simulink model "buckConverter"  (R2021a)
settings: Solver=VariableStepAuto  StartTime=0.0  StopTime=1  RelTol=1e-3
model workspace (MAT data in the model file):
  C = Simulink.Parameter
  C.Value = 0.01
  C.DataType = 'double'
  C.Dimensions = [1 1]
  L = Simulink.Parameter
  L.Value = 0.01
  L.DataType = 'double'
  L.Dimensions = [1 1]
  R = Simulink.Parameter
  R.Value = 10
  R.DataType = 'double'
  R.Dimensions = [1 1]
  Vin = Simulink.Parameter
  Vin.Value = 100
  Vin.DataType = 'double'
  Vin.Dimensions = [1 1]
libraries: spsSeriesRLCBranchLib x3, spsCurrentMeasurementLib x2, spsDCVoltageSourceLib x1, spsDiodeLib x1, spsIGBTLib x1, spsVoltageMeasurementLib x1, spspowerguiLib x1
settings Model: Creator=User  LastModifiedBy=User

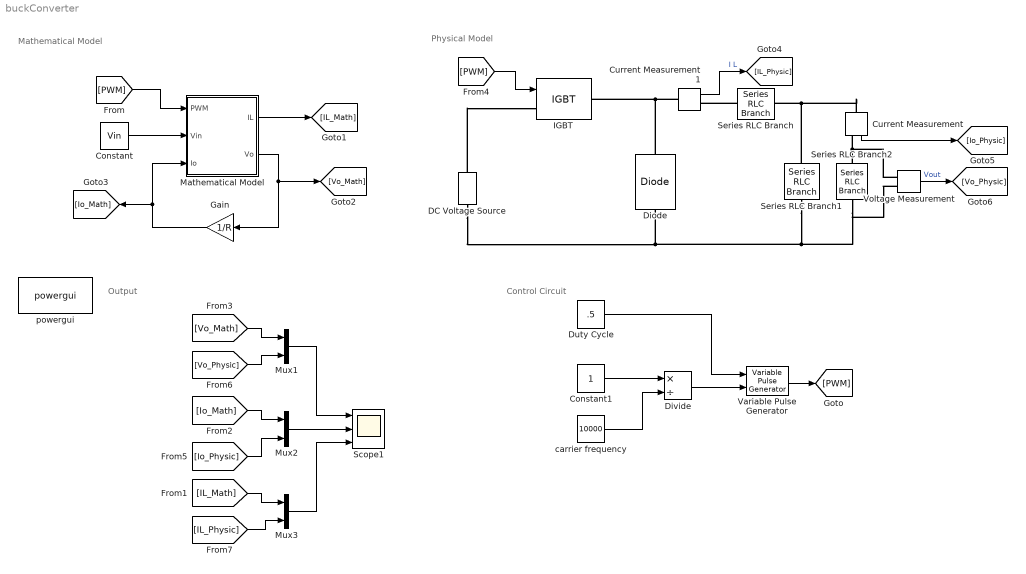
== system buckConverter ==
  note: Output
  note: Mathematical Model
  note: Physical Model
  note: Control Circuit
  Constant : Constant  Value=Vin
  Constant1 : Constant
  Current Measurement : spsCurrentMeasurementLib/Current Measurement  PhasorSimulation=off  OutputType=Complex  PSBequivalent=0
  Current Measurement1 : spsCurrentMeasurementLib/Current Measurement  PhasorSimulation=off  OutputType=Complex  PSBequivalent=0
  DC Voltage Source : spsDCVoltageSourceLib/DC Voltage Source  Amplitude=Vin  Measurements=None
  Diode : spsDiodeLib/Diode  Ron=0.001  Lon=0  Vf=0.8  IC=0  UseSnubber=0  Rs=500  Cs=250e-9  Measurements=off
  Divide : Product  Inputs=*/
  Duty Cycle : Constant  Value=.5
  Gain : Gain  Gain=1/R
  IGBT : spsIGBTLib/IGBT  Ron=0.001  Lon=0  Vf=1  Tf=1e-6  Tt=2e-6  IC=0  Rs=1e5  Cs=inf  Measurements=off
  Mathematical Model : Subsystem
  Mux1 : Mux  Inputs=2
  Mux2 : Mux  Inputs=2
  Mux3 : Mux  Inputs=2
  Scope1 : Scope  NumInputPorts=3
  Series RLC Branch : spsSeriesRLCBranchLib/Series RLC Branch  LConnTagsString=__new0  RConnTagsString=__new0  BranchType=L  Resistance=1  Inductance=L  SetiL0=off  InitialCurrent=0  Capacitance=1e-6  Setx0=off  InitialVoltage=0  Measurements=None
  Series RLC Branch1 : spsSeriesRLCBranchLib/Series RLC Branch  LConnTagsString=__new0  RConnTagsString=__new0  BranchType=C  Resistance=1  Inductance=1e-3  SetiL0=off  InitialCurrent=0  Capacitance=C  Setx0=off  InitialVoltage=0  Measurements=None
  Series RLC Branch2 : spsSeriesRLCBranchLib/Series RLC Branch  LConnTagsString=__new0  RConnTagsString=__new0  BranchType=R  Resistance=R  Inductance=1e-3  SetiL0=off  InitialCurrent=0  Capacitance=1e-6  Setx0=off  InitialVoltage=0  Measurements=None
  Variable Pulse Generator : VariablePulseGenerator  SampleTime=0.1
  Voltage Measurement : spsVoltageMeasurementLib/Voltage Measurement  PhasorSimulation=off  OutputType=Complex  PSBequivalent=0
  carrier frequency : Constant  Value=10000
  powergui : spspowerguiLib/powergui  Priority=1  SimulationMode=Continuous  SampleTime=50e-6  frequency=60  Iterations=50  frequencyindice=0  Pbase=100e6  ErrMax=1e-4  UnitsV=kV  UnitsW=MW  buscounter=0  FunctionMessages=off  echomessages=off  EnableUseOfTLC=off  CurrentSourceSwitches=off  DisableSnubberDevices=off  DisableRonSwitches=off  DisableVfSwitches=off  DisplayEquations=off  AutomaticDiscreteSolvers=off  SolverType=Tustin/Backward Euler (TBE)  Interpol=off  ExternalGateDelay=off  methode=off  Ts=100  x0status=blocks  SPID=on  SwTol=0  HookPort=off  NonlinearTolerance=1e-4  nMaxIteration=100  ContinueOnMaxIteration=off  RestoreLinks=warning  ResistiveCurrentMeasurement=off  Frange=[0:2:500]  Ylog=off  Xlog=on  ShowGrid=off  save=off  variable=ZData  structure=0  ZoomFFT=off  StartTime=0.0  cycles=1  DisplayStyle=1  fundamental=60  FreqAxis=off  MaxFrequency=1000  frequencyindicesteady=1  RmsSteady=1  display=off
  wires:
  Variable Pulse Generator/1 -> [PWM]
  Duty Cycle/1 -> Variable Pulse Generator/1
  Divide/1 -> Variable Pulse Generator/2
  Constant1/1 -> Divide/1
  carrier frequency/1 -> Divide/2
  [PWM] -> Mathematical Model/1(PWM)
  Constant/1 -> Mathematical Model/2(Vin)
  Mathematical Model/2(Vo) -> [Vo_Math], Gain/1
  Gain/1 -> [Io_Math], Mathematical Model/3(Io)
  Mathematical Model/1(IL) -> [IL_Math]
  Mux1/1 -> Scope1/1
  Mux2/1 -> Scope1/2
  Mux3/1 -> Scope1/3
  [Io_Math] -> Mux2/1
  [Vo_Math] -> Mux1/1
  [IL_Math] -> Mux3/1
  Current Measurement1/1 -> [IL_Physic]  "I L"
  Current Measurement/1 -> [Io_Physic]
  Voltage Measurement/1 -> [Vo_Physic]  "Vout"
  [Vo_Physic] -> Mux1/2
  [Io_Physic] -> Mux2/2
  [IL_Physic] -> Mux3/2
  [PWM] -> IGBT/1
  connections:
  DC Voltage Source/RConn1 -- IGBT/LConn1
  DC Voltage Source/LConn1 -- Diode/LConn1 -- Voltage Measurement/LConn2 -- Series RLC Branch2/RConn1 -- Series RLC Branch1/RConn1
  Series RLC Branch2/LConn1 -- Voltage Measurement/LConn1 -- Current Measurement/RConn1
  Current Measurement/LConn1 -- Series RLC Branch1/LConn1 -- Series RLC Branch/RConn1
  Series RLC Branch/LConn1 -- Current Measurement1/RConn1
  Diode/RConn1 -- Current Measurement1/LConn1 -- IGBT/RConn1

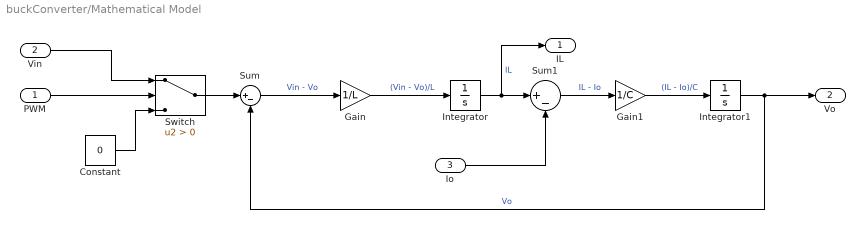
== system buckConverter/Mathematical Model ==
  PWM : Inport
  Vin : Inport  Port=2
  Io : Inport  Port=3
  Constant : Constant  Value=0
  Gain : Gain  Gain=1/L
  Gain1 : Gain  Gain=1/C
  Integrator : Integrator
  Integrator1 : Integrator
  Sum : Sum  Inputs=|+-
  Sum1 : Sum  Inputs=|+-
  Switch : Switch  Criteria=u2 > Threshold
  IL : Outport
  Vo : Outport  Port=2
  wires:
  Integrator/1 -> IL/1, Sum1/1  "IL"
  Vin/1 -> Switch/1
  Gain1/1 -> Integrator1/1  "(IL - Io)/C"
  Integrator1/1 -> Vo/1, Sum/2  "Vo"
  PWM/1 -> Switch/2
  Sum/1 -> Gain/1  "Vin - Vo"
  Switch/1 -> Sum/1
  Constant/1 -> Switch/3
  Gain/1 -> Integrator/1  "(Vin - Vo)/L"
  Sum1/1 -> Gain1/1  "IL - Io"
  Io/1 -> Sum1/2
